simulink model "Lab4_SystemType"  (R2016a)
settings: Solver=VariableStepAuto  StartTime=0.0  StopTime=10  MaxStep=.001  RelTol=1e-3
libraries: simulink x3
settings Model: Creator=jordan  LastModifiedBy=jordan

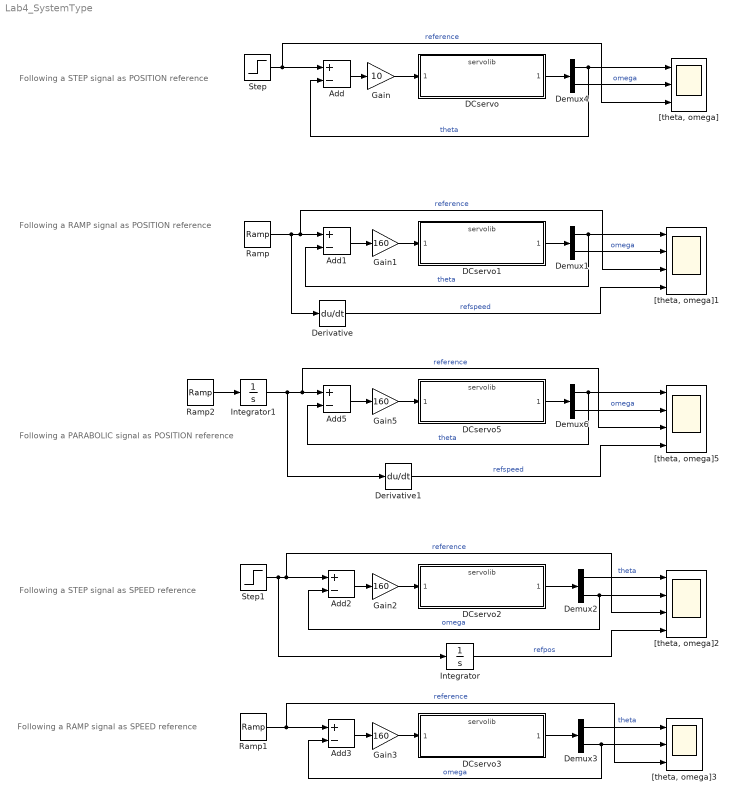
== system Lab4_SystemType ==
  note: Following a RAMP signal as
      | POSITION reference
  note: Following a STEP signal as
      | POSITION reference
  note: Following a PARABOLIC signal as
      | POSITION reference
  note: Following a STEP signal as
      | SPEED reference
  note: Following a RAMP signal as
      | SPEED reference
  Add{,1..3,5} (5 alike) : Sum  Inputs=+-
  DCservo{,1..3,5} (5 alike) : ModelReference  ModelNameDialog=servolib.slx  SimulationMode=Normal  ModelReferenceVersion=1.77
  Demux{1..4,6} (5 alike) : Demux  Outputs=2
  Derivative : Derivative
  Derivative1 : Derivative
  Gain : Gain  Gain=10
  Gain{1..3,5} (4 alike) : Gain  Gain=160
  Integrator : Integrator
  Integrator1 : Integrator
  Ramp : simulink/Sources/Ramp  slope=1  start=0  X0=0
  Ramp1 : simulink/Sources/Ramp  slope=.25  start=0  X0=0
  Ramp2 : simulink/Sources/Ramp  slope=1  start=0  X0=0
  Step : Step  SampleTime=0
  Step1 : Step  SampleTime=0
  "[theta, omega]" : Scope  NumInputPorts=3
  "[theta, omega]1" : Scope  NumInputPorts=4
  "[theta, omega]2" : Scope  NumInputPorts=4
  "[theta, omega]3" : Scope  NumInputPorts=3
  "[theta, omega]5" : Scope  NumInputPorts=4
  wires:
  Demux4/1 -> "[theta, omega]"/1, Add/2  "theta"
  Demux4/2 -> "[theta, omega]"/2  "omega"
  Add/1 -> Gain/1
  Gain/1 -> DCservo/1
  Step/1 -> "[theta, omega]"/3, Add/1  "reference"
  DCservo/1 -> Demux4/1
  Demux1/1 -> "[theta, omega]1"/1, Add1/2  "theta"
  Demux1/2 -> "[theta, omega]1"/2  "omega"
  Add1/1 -> Gain1/1
  Gain1/1 -> DCservo1/1
  Ramp/1 -> "[theta, omega]1"/3, Add1/1, Derivative/1  "reference"
  DCservo1/1 -> Demux1/1
  Demux2/1 -> "[theta, omega]2"/1  "theta"
  Demux2/2 -> "[theta, omega]2"/2, Add2/2  "omega"
  Add2/1 -> Gain2/1
  Gain2/1 -> DCservo2/1
  Step1/1 -> Integrator/1, "[theta, omega]2"/3, Add2/1  "reference"
  DCservo2/1 -> Demux2/1
  Demux3/1 -> "[theta, omega]3"/1  "theta"
  Demux3/2 -> "[theta, omega]3"/2, Add3/2  "omega"
  Add3/1 -> Gain3/1
  Gain3/1 -> DCservo3/1
  Ramp1/1 -> "[theta, omega]3"/3, Add3/1  "reference"
  DCservo3/1 -> Demux3/1
  Derivative/1 -> "[theta, omega]1"/4  "refspeed"
  Integrator/1 -> "[theta, omega]2"/4  "refpos"
  Demux6/1 -> "[theta, omega]5"/1, Add5/2  "theta"
  Demux6/2 -> "[theta, omega]5"/2  "omega"
  Add5/1 -> Gain5/1
  Gain5/1 -> DCservo5/1
  Ramp2/1 -> Integrator1/1
  DCservo5/1 -> Demux6/1
  Derivative1/1 -> "[theta, omega]5"/4  "refspeed"
  Integrator1/1 -> Derivative1/1, "[theta, omega]5"/3, Add5/1  "reference"
